simulink model "states_one"  (R2022b)
settings: Solver=FixedStepAuto  StartTime=0.0  StopTime=10.0  FixedStep=1e-3  RelTol=1e-3
settings Model: Creator=asolland  LastModifiedBy=asolland
settings OptimizationCC: DefaultParameterBehavior=Inlined  ReuseModelBlockBuffer=on  EnhancedBackFolding=on  PassReuseOutputArgsAs=Individual arguments  OptimizeBlockOrder=speed  DifferentSizesBufferReuse=on  OptimizationCustomize=off  EfficientTunableParamExpr=on
settings DebuggingCC: ParameterTunabilityLossMsg=error
settings HardwareCC: TargetBitPerLong=64  TargetBitPerPointer=64  TargetBitPerSizeT=64  TargetBitPerPtrDiffT=64  TargetLongLongMode=on  TargetIntDivRoundTo=Zero  TargetEndianess=LittleEndian  TargetWordSize=64  TargetHWDeviceType=MATLAB Host  ProdEqTarget=off
settings SFSimCC: MATLABDynamicMemAlloc=off
settings RTWCC: Description=Embedded Coder (host-based shared library target)  SystemTargetFile=sim_pandas.tlc  TemplateMakefile=ert_default_tmf  GPUComputeCapability=5.0
settings CodeAppCC: ForceParamTrailComments=on  OperatorAnnotations=on  SimulinkDataObjDesc=on  SFDataObjDesc=on  InsertBlockDesc=on
settings STFCustomTargetCC: TargetLangStandard=C99 (ISO)  MultiwordLength=256  GenerateSampleERTMain=on  ParMdlRefBuildCompliant=on  CompOptLevelCompliant=on  CombineOutputUpdateFcns=on  ERTCustomFileBanners=on  CodeInterfacePackaging=Reusable function  SupportContinuousTime=off  SupportNonInlinedSFcns=off  RemoveResetFunc=on  MATLABClassNameForMDSCustomization=Simulink.SoftwareTarget.ERTCustomization  ModelStepFunctionPrototypeControlCompliant=on  UseToolchainInfoCompliant=on  SystemTargetFile=sim_pandas.tlc
settings ERTTargetCC: TargetLangStandard=C99 (ISO)  GenerateSampleERTMain=on  ConcurrentExecutionCompliant=off  CodeInterfacePackaging=Reusable function  CPPClassGenCompliant=off  InlinedParameterPlacement=NonHierarchical  RootIOFormat=Part of model data structure  ERTCustomFileTemplate=example_file_process.tlc
settings ConfigComp: CovBoundaryAbsTol=1.0e-5

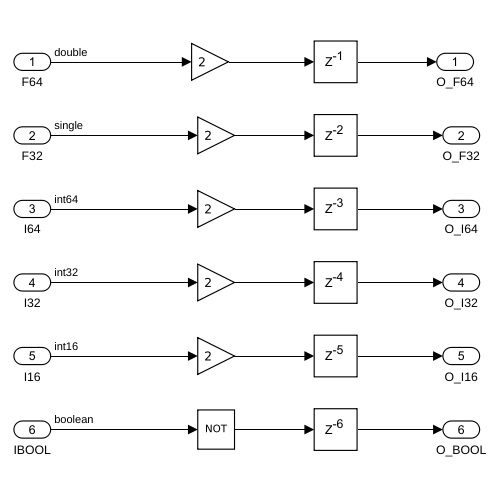
[thumbnail: Simulink's stored preview of the top-level diagram]
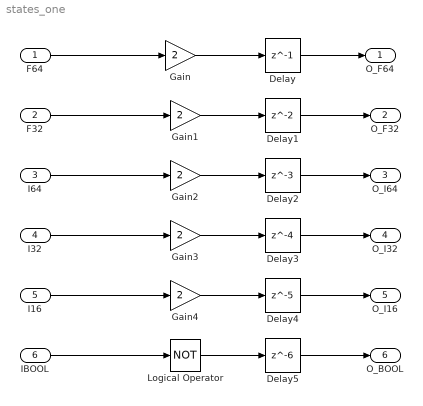
== system states_one ==
  F64 : Inport  OutDataTypeStr=double
  F32 : Inport  Port=2  OutDataTypeStr=single
  I64 : Inport  Port=3  OutDataTypeStr=int64
  I32 : Inport  Port=4  OutDataTypeStr=int32
  I16 : Inport  Port=5  OutDataTypeStr=int16
  IBOOL : Inport  Port=6  OutDataTypeStr=boolean
  Delay : Delay  DelayLength=1
  Delay1 : Delay
  Delay2 : Delay  DelayLength=3
  Delay3 : Delay  DelayLength=4
  Delay4 : Delay  DelayLength=5
  Delay5 : Delay  DelayLength=6
  Gain{,1..4} (5 alike) : Gain  Gain=2  OutDataTypeStr=Inherit: Same as input  ParamDataTypeStr=Inherit: Same as input
  Logical Operator : Logic  Operator=NOT  AllPortsSameDT=off  OutDataTypeStr=boolean
  O_F64 : Outport
  O_F32 : Outport  Port=2
  O_I64 : Outport  Port=3
  O_I32 : Outport  Port=4
  O_I16 : Outport  Port=5
  O_BOOL : Outport  Port=6
  wires:
  F64/1 -> Gain/1
  Gain/1 -> Delay/1
  Gain1/1 -> Delay1/1
  F32/1 -> Gain1/1
  Gain2/1 -> Delay2/1
  Gain3/1 -> Delay3/1
  Gain4/1 -> Delay4/1
  I64/1 -> Gain2/1
  I32/1 -> Gain3/1
  I16/1 -> Gain4/1
  IBOOL/1 -> Logical Operator/1
  Logical Operator/1 -> Delay5/1
  Delay/1 -> O_F64/1
  Delay1/1 -> O_F32/1
  Delay2/1 -> O_I64/1
  Delay3/1 -> O_I32/1
  Delay4/1 -> O_I16/1
  Delay5/1 -> O_BOOL/1
